simulink library "csc_cam_camera_system_lib"  (R2014b)
settings: Solver=ode45  SolverMode=SingleTasking  StartTime=0.0  StopTime=10.0  RelTol=1e-3
values from neighbouring files (symbols this model uses):
  cam_process_pair_counter = round(cam_process_delta_t/sim_time_step_size)    [csc_cam_camera_system_prep.m]
  cam_take_image_counter = round(cam_image_delta_t/sim_time_step_size)    [csc_cam_camera_system_prep.m]
  cam_use_meme_flag = csc_cam_establish_meme_contact(cam_attempt_to_use_meme_flag, meme_ip, meme_port)    [csc_cam_camera_system_prep.m]    (also in csc_cam_establish_meme_contact.m = 0)
undefined symbols (not defined in the file or in its folder): KF_DT, pwr_sta_on_state
libraries: simulink x2, csc_cmg_camera_geometry_lib x2, util_info_lib x1, csc_fdm_feature_detection_matching_lib x1, csu_kfd_orb_feature_matching_lib x1
settings Model: Creator=hcannon  LastModifiedBy=mstewart

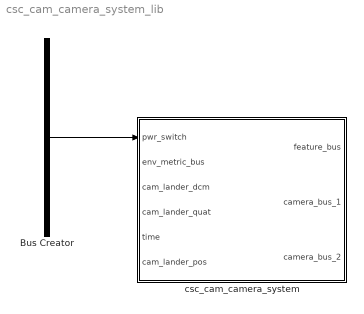
== system csc_cam_camera_system_lib ==
  Bus Creator : BusCreator  Inputs=10
  csc_cam_camera_system : Subsystem  SystemSampleTime=KF_DT
  wires:
  ? -> Bus Creator/10  "grv_gravity_acc_eci"
  ? -> Bus Creator/1  "rrd_alpha_body_in_eci"
  ? -> Bus Creator/2  "rrk_rate_body_eci_body"
  ? -> Bus Creator/3  "rrk_q_body_from_eci"
  ? -> Bus Creator/4  "rrk_euler_zyx_rot_deg"
  ? -> Bus Creator/5  "rtd_acc_body_in_eci"
  ? -> Bus Creator/6  "rtk_vel_eci"
  ? -> Bus Creator/7  "rtk_pos_eci"
  ? -> Bus Creator/8
  ? -> Bus Creator/9
  Bus Creator/1 -> csc_cam_camera_system/1(pwr_switch)

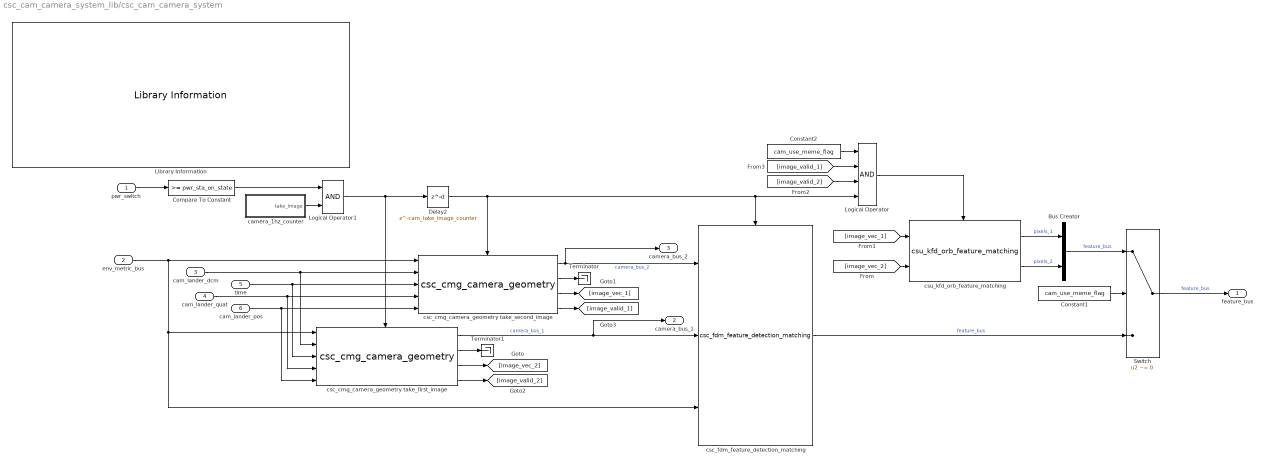
== system csc_cam_camera_system_lib/csc_cam_camera_system ==
  pwr_switch : Inport
  env_metric_bus : Inport  Port=2
  cam_lander_dcm : Inport  Port=3
  cam_lander_quat : Inport  Port=4
  time : Inport  Port=5
  cam_lander_pos : Inport  Port=6
  Bus Creator : BusCreator  Inputs=2
  Compare To Constant : simulink/Logic and Bit Operations/Compare To Constant  relop=>=  const=pwr_sta_on_state  OutDataTypeStr=boolean
  Constant1 : Constant  Value=cam_use_meme_flag
  Constant2 : Constant  Value=cam_use_meme_flag
  Delay2 : Delay  DelayLength=cam_take_image_counter
  Library Information : util_info_lib/Library Information  owner='NONE'
  Logical Operator : Logic  Inputs=4  AllPortsSameDT=off  OutDataTypeStr=boolean
  Logical Operator1 : Logic  AllPortsSameDT=off  OutDataTypeStr=boolean
  Switch : Switch  Criteria=u2 ~= 0
  Terminator : Terminator
  Terminator1 : Terminator
  camera_1hz_counter : Subsystem  TreatAsAtomicUnit=on
  csc_cmg_camera_geometry take_first_image : csc_cmg_camera_geometry_lib/csc_cmg_camera_geometry
  csc_cmg_camera_geometry take_second_image : csc_cmg_camera_geometry_lib/csc_cmg_camera_geometry
  csc_fdm_feature_detection_matching : csc_fdm_feature_detection_matching_lib/csc_fdm_feature_detection_matching
  csu_kfd_orb_feature_matching : csu_kfd_orb_feature_matching_lib/csu_kfd_orb_feature_matching  size=cam_kir_image_size
  feature_bus : Outport
  camera_bus_1 : Outport  Port=2
  camera_bus_2 : Outport  Port=3
  wires:
  Compare To Constant/1 -> Logical Operator1/1
  camera_1hz_counter/1(take_image) -> Logical Operator1/2
  pwr_switch/1 -> Compare To Constant/1
  Logical Operator1/1 -> Delay2/1, csc_cmg_camera_geometry take_first_image/Enable
  cam_lander_pos/1 -> csc_cmg_camera_geometry take_second_image/5, csc_cmg_camera_geometry take_first_image/5
  Constant1/1 -> Switch/2
  csc_fdm_feature_detection_matching/1 -> Switch/3  "feature_bus"
  Switch/1 -> feature_bus/1  "feature_bus"
  Bus Creator/1 -> Switch/1  "feature_bus"
  csu_kfd_orb_feature_matching/1 -> Bus Creator/1  "pixels_1"
  csu_kfd_orb_feature_matching/2 -> Bus Creator/2  "pixels_2"
  Logical Operator/1 -> csu_kfd_orb_feature_matching/Enable
  [image_vec_2] -> csu_kfd_orb_feature_matching/2
  [image_vec_1] -> csu_kfd_orb_feature_matching/1
  time/1 -> csc_cmg_camera_geometry take_first_image/3, csc_cmg_camera_geometry take_second_image/3
  cam_lander_quat/1 -> csc_cmg_camera_geometry take_second_image/4, csc_cmg_camera_geometry take_first_image/4
  cam_lander_dcm/1 -> csc_cmg_camera_geometry take_first_image/2, csc_cmg_camera_geometry take_second_image/2
  csc_cmg_camera_geometry take_second_image/1 -> csc_fdm_feature_detection_matching/1, camera_bus_2/1  "camera_bus_2"
  env_metric_bus/1 -> csc_cmg_camera_geometry take_second_image/1, csc_fdm_feature_detection_matching/3, csc_cmg_camera_geometry take_first_image/1
  Delay2/1 -> Logical Operator/4, csc_fdm_feature_detection_matching/Enable, csc_cmg_camera_geometry take_second_image/Enable
  csc_cmg_camera_geometry take_first_image/1 -> csc_fdm_feature_detection_matching/2, camera_bus_1/1  "camera_bus_1"
  [image_valid_1] -> Logical Operator/2
  [image_valid_2] -> Logical Operator/3
  Constant2/1 -> Logical Operator/1
  csc_cmg_camera_geometry take_second_image/4 -> [image_valid_1]
  csc_cmg_camera_geometry take_second_image/3 -> [image_vec_1]
  csc_cmg_camera_geometry take_second_image/2 -> Terminator/1
  csc_cmg_camera_geometry take_first_image/4 -> [image_valid_2]
  csc_cmg_camera_geometry take_first_image/3 -> [image_vec_2]
  csc_cmg_camera_geometry take_first_image/2 -> Terminator1/1

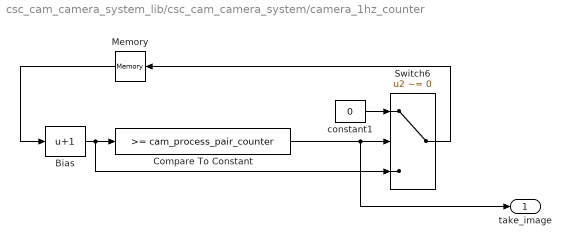
== system csc_cam_camera_system_lib/csc_cam_camera_system/camera_1hz_counter ==
  Bias : Bias  Bias=1
  Compare To Constant : simulink/Logic and Bit Operations/Compare To Constant  relop=>=  const=cam_process_pair_counter  OutDataTypeStr=uint8
  Memory : Memory  X0=cam_process_pair_counter  InheritSampleTime=on
  Switch6 : Switch  Criteria=u2 ~= 0  InputSameDT=on
  constant1 : Constant  Value=0
  take_image : Outport
  wires:
  Memory/1 -> Bias/1
  Switch6/1 -> Memory/1
  Compare To Constant/1 -> take_image/1, Switch6/2
  Bias/1 -> Switch6/3, Compare To Constant/1
  constant1/1 -> Switch6/1
